simulink model "Stand_DCM_Simulation"  (R2024a)
settings: Solver=VariableStepAuto  StartTime=0.0  StopTime=10  RelTol=1e-3
settings Model: Creator=adminLab  LastModifiedBy=adminLab

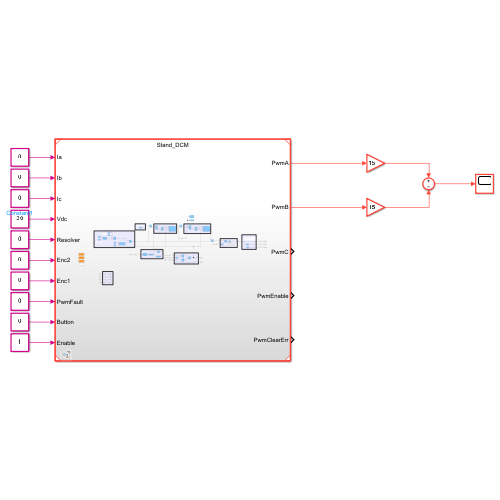
[thumbnail: Simulink's stored preview of the top-level diagram]
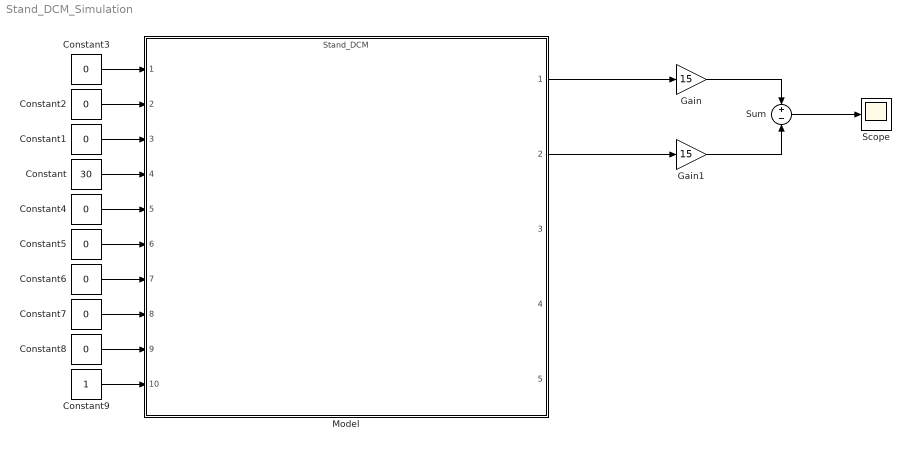
== system Stand_DCM_Simulation ==
  Constant : Constant  Value=30
  Constant{1..8} (8 alike) : Constant  Value=0
  Constant9 : Constant
  Gain : Gain  Gain=15
  Gain1 : Gain  Gain=15
  Model : ModelReference  ModelNameDialog=Stand_DCM.slx  SimulationMode=Normal  ModelReferenceVersion=11.49
  Scope : Scope
  Sum : Sum  Inputs=+|-
  wires:
  Constant/1 -> Model/4
  Model/2 -> Gain1/1
  Model/1 -> Gain/1
  Gain/1 -> Sum/1
  Gain1/1 -> Sum/2
  Sum/1 -> Scope/1
  Constant3/1 -> Model/1
  Constant2/1 -> Model/2
  Constant1/1 -> Model/3
  Constant9/1 -> Model/10
  Constant4/1 -> Model/5
  Constant5/1 -> Model/6
  Constant6/1 -> Model/7
  Constant7/1 -> Model/8
  Constant8/1 -> Model/9
